simulink model "MotorParameterEstimation"  (R2019b)
settings: Solver=VariableStepAuto  StartTime=0.0  StopTime=10  MaxStep=1e-4  RelTol=1e-3
PreLoadFcn:
  | modelDir = fileparts(get_param(bdroot, 'FileName'));
  | addpath(fullfile(modelDir,'../Parameters'));
  | addpath(fullfile(modelDir,'subsystems'));
  | 
  | Parameters_Model
  | Parameters_Simulation
  | Parameters_Controller
InitFcn:
  | Parameters_Model
  | Parameters_Simulation
  | Parameters_Controller
libraries: simulink x3
settings Model: Creator=Thomas  LastModifiedBy=thomas.jespersen
settings DataIOCC: ReturnWorkspaceOutputs=off
settings DebuggingCC: ArithmeticOperatorsInVariantConditions=warning
settings SFSimCC: SimUseLocalCustomCode=off  CustomCodeUndefinedFunction=UseInterfaceOnly
settings RTWCC: RTWUseLocalCustomCode=off

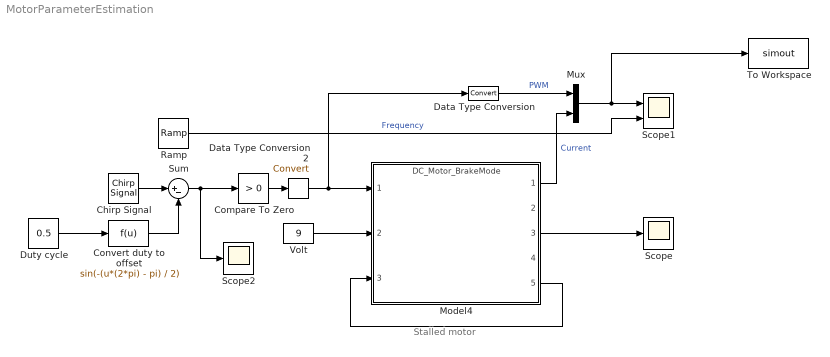
== system MotorParameterEstimation ==
  note: Stalled motor
  Chirp Signal : simulink/Sources/Chirp Signal  f1=100  T=10  f2=10000
  Compare To Zero : simulink/Logic and Bit Operations/Compare To Zero  relop=>  OutDataTypeStr=boolean
  Convert duty to offset : Fcn  Expr=sin(-(u*(2*pi) - pi) / 2)
  Data Type Conversion : DataTypeConversion
  Data Type Conversion2 : DataTypeConversion  RndMeth=Round
  Duty cycle : Constant  Value=0.5
  Model4 : ModelReference  ModelNameDialog=DC_Motor_BrakeMode  SimulationMode=Normal  ModelReferenceVersion=1.44
  Mux : Mux  Inputs=2
  Ramp : simulink/Sources/Ramp  slope=(10000-100)/10  start=0  InitialOutput=100
  Scope : Scope
  Scope1 : Scope  NumInputPorts=2
  Scope2 : Scope
  Sum : Sum  Inputs=|+-
  To Workspace : ToWorkspace  VariableName=simout  SaveFormat=Timeseries  SampleTime=-1
  Volt : Constant  Value=9
  wires:
  Volt/1 -> Model4/2
  Compare To Zero/1 -> Data Type Conversion2/1
  Model4/5 -> Model4/3
  Model4/1 -> Mux/2  "Current"
  Mux/1 -> To Workspace/1, Scope1/1
  Ramp/1 -> Scope1/2  "Frequency"
  Data Type Conversion/1 -> Mux/1  "PWM"
  Model4/3 -> Scope/1
  Chirp Signal/1 -> Sum/1
  Sum/1 -> Scope2/1, Compare To Zero/1
  Convert duty to offset/1 -> Sum/2
  Duty cycle/1 -> Convert duty to offset/1
  Data Type Conversion2/1 -> Data Type Conversion/1, Model4/1
